simulink model "Ex3"  (R2020a)
settings: Solver=VariableStepAuto  StartTime=0.0  StopTime=10.0  RelTol=1e-3
model workspace (MAT data in the model file):
  I = 1
  KD = 1
  KI = 1
  KP = 4
  MD = 2
  Ref = 1
  d = 1
settings Model: Creator=Pongsakorn  LastModifiedBy=Pongsakorn

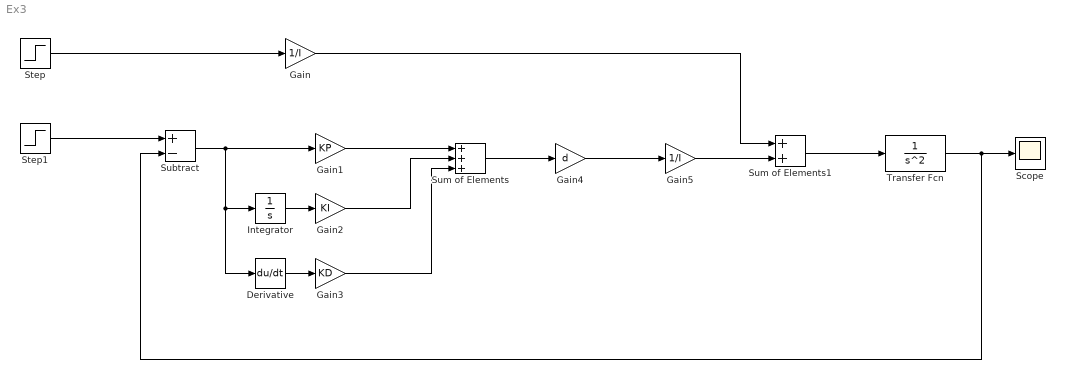
== system Ex3 ==
  Derivative : Derivative
  Gain : Gain  Gain=1/I
  Gain1 : Gain  Gain=KP
  Gain2 : Gain  Gain=KI
  Gain3 : Gain  Gain=KD
  Gain4 : Gain  Gain=d
  Gain5 : Gain  Gain=1/I
  Integrator : Integrator
  Scope : Scope
  Step : Step  After=MD  SampleTime=0
  Step1 : Step  After=Ref  SampleTime=0
  Subtract : Sum  Inputs=+-
  Sum of Elements : Sum  Inputs=+++  CollapseMode=Specified dimension  CollapseDim=3
  Sum of Elements1 : Sum  CollapseMode=Specified dimension  CollapseDim=3
  Transfer Fcn : TransferFcn  Denominator=[1 0 0]
  wires:
  Step/1 -> Gain/1
  Step1/1 -> Subtract/1
  Subtract/1 -> Derivative/1, Integrator/1, Gain1/1
  Integrator/1 -> Gain2/1
  Derivative/1 -> Gain3/1
  Gain1/1 -> Sum of Elements/1
  Gain2/1 -> Sum of Elements/2
  Gain3/1 -> Sum of Elements/3
  Gain/1 -> Sum of Elements1/1
  Gain5/1 -> Sum of Elements1/2
  Gain4/1 -> Gain5/1
  Sum of Elements/1 -> Gain4/1
  Sum of Elements1/1 -> Transfer Fcn/1
  Transfer Fcn/1 -> Subtract/2, Scope/1
